simulink model "sampleModel277"  (R2021b)
settings: Solver=VariableStepAuto  StartTime=0.0  StopTime=10.0  RelTol=1e-3
undefined symbols (not defined in the file or in its folder): Newton, Raphson
libraries: simulink x9, slpidlib x1
settings Model: Creator=user  LastModifiedBy=user

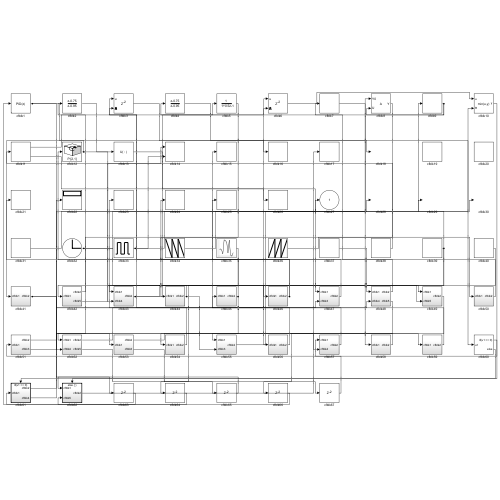
[thumbnail: Simulink's stored preview of the top-level diagram]
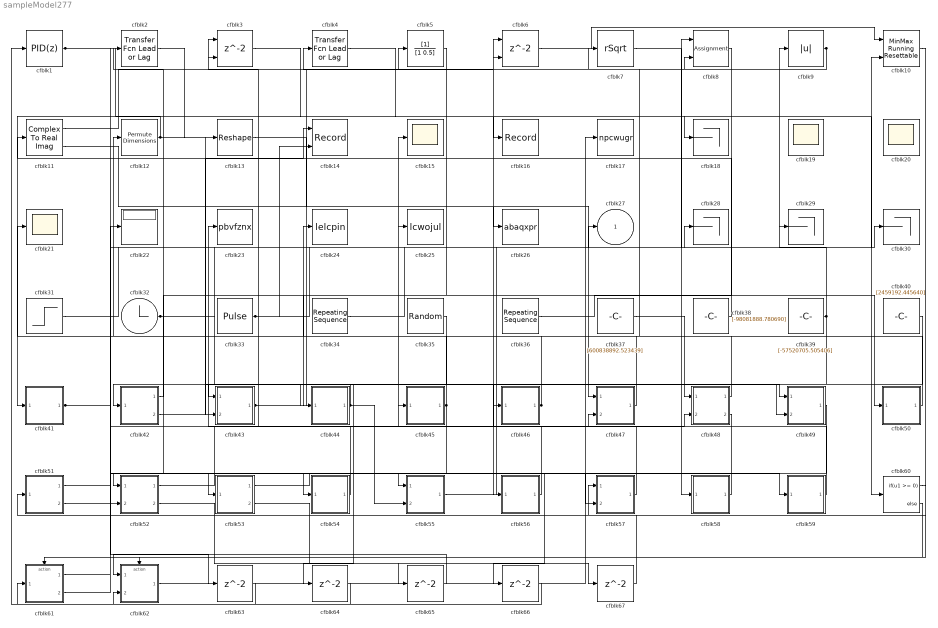
== system sampleModel277 ==
  cfblk1 : slpidlib/PID Controller  Controller=PID  Form=Parallel  TimeDomain=Discrete-time  UseExternalTs=off  SampleTime=1  IntegratorMethod=Forward Euler  FilterMethod=Forward Euler  ControllerParametersSource=internal  P=1  I=1  D=0  UseFilter=on  N=100  TunerSelectOption=Transfer Function Based (PID Tuner App)  InitialConditionSource=internal  InitialConditionForIntegrator=0  InitialConditionForFilter=0  DifferentiatorICPrevScaledInput=0  ExternalReset=none  TrackingMode=off  Kt=1  LimitOutput=off  SatLimitsSource=internal  UpperSaturationLimit=inf  LowerSaturationLimit=-inf  LinearizeAsGain=off  AntiWindupMode=none  Kb=1  POutMin=[]  POutMax=[]  IOutMin=[]  IOutMax=[]  DOutMin=[]  DOutMax=[]  NOutMin=[]  NOutMax=[]  SumOutMin=[]  SumOutMax=[]  SaturationOutMin=[]  SaturationOutMax=[]  PParamMin=[]  PParamMax=[]  IParamMin=[]  IParamMax=[]  DParamMin=[]  DParamMax=[]  NParamMin=[]  NParamMax=[]  KbParamMin=[]  KbParamMax=[]  KtParamMin=[]  KtParamMax=[]  KbOutMin=[]  KbOutMax=[]  KtOutMin=[]  KtOutMax=[]  IntegratorOutMin=[]  IntegratorOutMax=[]  FilterOutMin=[]  FilterOutMax=[]  SumI1OutMin=[]  SumI1OutMax=[]  SumI2OutMin=[]  SumI2OutMax=[]  SumI3OutMin=[]  SumI3OutMax=[]  SumI4OutMin=[]  SumI4OutMax=[]  SumDOutMin=[]  SumDOutMax=[]  DifferentiatorOutMin=[]  DifferentiatorOutMax=[]  FilterDiffOutCoefMin=[]  FilterDiffOutCoefMax=[]  ReciprocalOutMin=[]  ReciprocalOutMax=[]  SumDenOutMin=[]  SumDenOutMax=[]  SumNumOutMin=[]  SumNumOutMax=[]  DivideOutMin=[]  DivideOutMax=[]  UdiffTsProdOutMin=[]  UdiffTsProdOutMax=[]  NTsProdOutMin=[]  NTsProdOutMax=[]  UintegralTsProdOutMin=[]  UintegralTsProdOutMax=[]  UngainTsProdOutMin=[]  UngainTsProdOutMax=[]  IntegratorContinuousStateAttributes=''  IntegratorStateMustResolveToSignalObject=off  IntegratorRTWStateStorageClass=Auto  FilterContinuousStateAttributes=''  FilterStateMustResolveToSignalObject=off  FilterRTWStateStorageClass=Auto  ParallelPVariant=InternalParameters  IdealPVariant=Disabled  IVariant=InternalParameters  DVariant=InternalParameters  IntegratorVariant=Discrete  SatVariant=Disabled  AWVariant=Passthrough  PCopyVariant=Disabled  TRVariant=Disabled  FdbkBlocksVariant=Forward  IdealPFdbkVariant=Disabled  SatFdbkVariant=Disabled  DerivativeFilterVariant=ForwardEulerFilter  NVariant=InternalParameters  NCopyVariant=Disabled  FilterICVariant=InternalICsFilter  IntegratorICVariant=InternalICs  ExternalResetVariant=Disabled  TRSumVariant=Passthrough  SumFdbkVariant=Disabled  SumVariant=Sum_PID  TsampFilterVariant=InternalTs  TsampNgainVariant=Passthrough  TsampIntegralVariant=Passthrough  ExternalSaturationOutDataTypeStr=Inherit: Same as second input
  cfblk10 : simulink/Math Operations/MinMax Running Resettable  Function=min  vinit=0.0
  cfblk11 : ComplexToRealImag
  cfblk12 : PermuteDimensions
  cfblk13 : Reshape
  cfblk14 : Record  FileSettingsInternal="{\"entries\":[{\"content\":{\"excelSettings\":{\"content\":{},\"type\":\"Streamout.ExcelSettings\"}},\"type\":\"Streamout.FileSettingStorage\",\"uuid\":\"d8607e28-881b-4112-add2-e3f322c6c66a\"}],\"packageUris\":[\"http://schema.mathworks.com/mf0/streamout_blocks/R2020a\"],\"version\":\"1.0\"}"  Layout=[1 1]  SignalsInternal="{\"entries\":[{\"content\":{\"signals\":[{\"content\":{\"blockPath\":[\"sampleModel277/cfblk14\"],\"channel\":[],\"dimensions\":[1],\"domain\":\"sampleModel277/cfblk14\",\"lineColor\":\"#a2142f\",\"plots\":[1],\"port\":1,\"sid\":[\"\"],\"signalID\":11589,\"signalName\":\"cfblk42:2\"},\"type\":\"RecordBlkView.Signal\",\"uuid\":\"b47615fb-d819-4e60-bc98-0c25ee9ba6d9\"},{\"content\":{\"blockPath\":[\"sampleModel277/cfblk14\"],\"channel\":[],\"dimensions\":[1],\"domain\":\"sampleModel277/cfblk14\",\"lineColor\":\"#139fff\",\"plots\":[1],\"port\":2,\"sid\":[\"\"],\"signalID\":11593,\"signalName\":\"cfblk33\"},\"type\":\"RecordBlkView.Signal\",\"uuid\":\"1de72bfb-52b8-4dac-a285-8f2b21a8e79d\"}]},\"type\":\"RecordBlkView.InputSignals\",\"uuid\":\"f8287ad3-c409-4800-adb5-27c45d527277\"}],\"packageUris\":[\"http://schema.mathworks.com/mf0/streamout_blocks/R2020a\"],\"version\":\"1.0\"}"  VisualizationBindings="{\"xyplotplugin\":{\"info\":[{\"series\":[{\"bindingParametersList\":[{\"parameter\":\"X-Axis\",\"signalID\":11589,\"signalName\":\"cfblk42:2\"},{\"parameter\":\"Y-Axis\",\"signalID\":11593,\"signalName\":\"cfblk33\"}],\"seriesID\":22106}],\"subplotID\":1}]}}"  CompatibilityTag=XY
  cfblk{15,19..21} (4 alike) : Scope
      cfblk19 settings: Floating=on
      cfblk20 settings: Floating=on
  cfblk16 : Record  FileSettingsInternal="{\"entries\":[{\"content\":{\"excelSettings\":{\"content\":{},\"type\":\"Streamout.ExcelSettings\"}},\"type\":\"Streamout.FileSettingStorage\",\"uuid\":\"0defbab6-1f19-424a-8477-c9e0ae50d269\"}],\"packageUris\":[\"http://schema.mathworks.com/mf0/streamout_blocks/R2020a\"],\"version\":\"1.0\"}"  SignalsInternal="{\"entries\":[{\"content\":{\"signals\":[{\"content\":{\"blockPath\":[\"sampleModel277/cfblk16\"],\"channel\":[],\"dimensions\":[1],\"domain\":\"sampleModel277/cfblk16\",\"lineColor\":\"#ff13a6\",\"plots\":[1],\"port\":1,\"sid\":[\"\"],\"signalID\":11597,\"signalName\":\"cfblk4\"},\"type\":\"RecordBlkView.Signal\",\"uuid\":\"1bcd9140-bb26-4ac9-91fa-95d908c78e84\"}]},\"type\":\"RecordBlkView.InputSignals\",\"uuid\":\"defb70cb-bd16-40b5-b6bd-1390d4c46c9b\"}],\"packageUris\":[\"http://schema.mathworks.com/mf0/streamout_blocks/R2020a\"],\"version\":\"1.0\"}"  VisualizationBindings="{\"sparklinesplugin\":{\"info\":[{\"bindingParametersList\":[],\"subplotID\":1}]}}"
  cfblk17 : ToWorkspace  VariableName=npcwugr  SaveFormat=Timeseries  SampleTime=-1
  cfblk{18,28..30} (4 alike) : Terminator
  cfblk2 : simulink/Discrete/Transfer Fcn Lead or Lag  PoleZ=0.95  ZeroZ=0.75  ICPrevOutput=0.0  ICPrevInput=0.0  DoSatur=off
      settings: SourceProductBaseCode=SL
  cfblk22 : Display
  cfblk23 : ToWorkspace  VariableName=pbvfznx  SaveFormat=Timeseries  SampleTime=-1
  cfblk24 : ToWorkspace  VariableName=lelcpin  SaveFormat=Timeseries  SampleTime=-1
  cfblk25 : ToWorkspace  VariableName=lcwojul  SaveFormat=Timeseries  SampleTime=-1
  cfblk26 : ToWorkspace  VariableName=abaqxpr  SaveFormat=Timeseries  SampleTime=-1
  cfblk3 : Delay  ShowEnablePort=on  SampleTime=1
      settings: InputPortMap=u0,e6
  cfblk31 : Step  Time=[8.000000]  Before=[446463938.940036]  After=[511590212.511346]  SampleTime=0
  cfblk32 : Clock
  cfblk33 : DiscretePulseGenerator  PulseType=Time based  Amplitude=[-336989697.738639]  Period=[82161498.785014]  PulseWidth=5  PhaseDelay=[6.000000]
  cfblk34 : simulink/Sources/Repeating Sequence  rep_seq_t=[0 2]  rep_seq_y=[583198754.923959, 299174869.221675]
  cfblk35 : RandomNumber  Mean=[14216.609925]  Variance=[79975.789287]  Seed=[438589470.000000]  SampleTime=0.1
  cfblk36 : simulink/Sources/Repeating Sequence  rep_seq_t=[0 2]  rep_seq_y=[305355629.704931, 356437179.098536]
  cfblk37 : Constant  Value=[600838892.523439]  SampleTime=1
  cfblk38 : Constant  Value=[-98081888.780690]  SampleTime=1
  cfblk39 : Constant  Value=[-57520705.505406]  SampleTime=1
  cfblk4 : simulink/Discrete/Transfer Fcn Lead or Lag  PoleZ=0.95  ZeroZ=0.75  ICPrevOutput=0.0  ICPrevInput=0.0  DoSatur=off
      settings: SourceProductBaseCode=SL
  cfblk40 : Constant  Value=[2459192.445640]  SampleTime=1
  cfblk41 : Subsystem
  cfblk42 : Subsystem
  cfblk43 : Subsystem
  cfblk44 : Subsystem
  cfblk45 : Subsystem
  cfblk46 : Subsystem
  cfblk47 : Subsystem
  cfblk48 : Subsystem
  cfblk49 : Subsystem
  cfblk5 : DiscreteFilter  SampleTime=1
  cfblk50 : Subsystem
  cfblk51 : Subsystem
  cfblk52 : Subsystem
  cfblk53 : Subsystem
  cfblk54 : Subsystem
  cfblk55 : Subsystem
  cfblk56 : Subsystem
  cfblk57 : Subsystem
  cfblk58 : Subsystem
  cfblk59 : Subsystem
  cfblk6 : Delay  ShowEnablePort=on  SampleTime=1
      settings: InputPortMap=u0,e6
  cfblk60 : If  IfExpression=u1 >= 0  SampleTime=1
  cfblk61 : Subsystem  TreatAsAtomicUnit=on
  cfblk62 : Subsystem  TreatAsAtomicUnit=on
  cfblk{63..67} (5 alike) : Delay  SampleTime=1
  cfblk7 : Sqrt  Operator=rSqrt  AlgorithmType=Newton-Raphson  SaturateOnIntegerOverflow=on
  cfblk8 : Assignment  DiagnosticForDimensions=Warning  IndexOptions=Index vector (dialog)  Indices=1  OutputSizes=1
  cfblk9 : Abs
  cfblk27 : Outport
  wires:
  cfblk53/1(cfblk2) -> cfblk59/1(cfblk1)
  cfblk48/1(cfblk2) -> cfblk12/1
  cfblk44/1(cfblk2) -> cfblk42/1(cfblk1), cfblk55/2(cfblk3)
  cfblk2/1 -> cfblk13/1
  cfblk54/1(cfblk2) -> cfblk23/1
  cfblk36/1 -> cfblk50/1(cfblk1)
  cfblk6/1 -> cfblk10/1
  cfblk9/1 -> cfblk4/1, cfblk8/2
  cfblk10/1 -> cfblk57/1(cfblk1)
  cfblk12/1 -> cfblk41/1(cfblk1), cfblk49/2(cfblk5)
  cfblk11/1 -> cfblk6/1
  cfblk43/1(cfblk2) -> cfblk5/1, cfblk49/1(cfblk1)
  cfblk31/1 -> cfblk9/1
  cfblk58/1(cfblk2) -> cfblk55/1(cfblk1)
  cfblk40/1 -> cfblk43/1(cfblk1)
  cfblk11/2 -> cfblk47/1(cfblk1)
  cfblk52/1(cfblk2) -> cfblk6/2
  cfblk38/1 -> cfblk11/1
  cfblk35/1 -> cfblk43/2(cfblk4)
  cfblk1/1 -> cfblk60/1, cfblk57/2(cfblk4)
  cfblk13/1 -> cfblk26/1
  cfblk39/1 -> cfblk29/1, cfblk54/1(cfblk1), cfblk46/1(cfblk1)
  cfblk55/1(cfblk2) -> cfblk28/1
  cfblk62/1(cfblk2) -> cfblk17/1
  cfblk3/1 -> cfblk18/1
  cfblk59/1(cfblk2) -> cfblk15/1
  cfblk34/1 -> cfblk30/1
  cfblk33/1 -> cfblk10/2, cfblk14/2
  cfblk50/1(cfblk2) -> cfblk7/1
  cfblk41/1(cfblk2) -> cfblk47/2(cfblk3), cfblk63/1
  cfblk42/1(cfblk2) -> cfblk2/1
  cfblk45/1(cfblk2) -> cfblk25/1, cfblk64/1
  cfblk57/1(cfblk2) -> cfblk45/1(cfblk1)
  cfblk37/1 -> cfblk48/1(cfblk1)
  cfblk32/1 -> cfblk56/1(cfblk1), cfblk8/1
  cfblk8/1 -> cfblk44/1(cfblk1)
  cfblk5/1 -> cfblk52/1(cfblk1)
  cfblk49/1(cfblk2) -> cfblk52/2(cfblk4)
  cfblk7/1 -> cfblk58/1(cfblk1)
  cfblk47/1(cfblk2) -> cfblk24/1
  cfblk46/1(cfblk2) -> cfblk21/1, cfblk3/2
  cfblk56/1(cfblk2) -> cfblk3/1
  cfblk4/1 -> cfblk16/1
  cfblk51/1(cfblk2) -> cfblk53/1(cfblk1)
  cfblk42/2(cfblk5) -> cfblk14/1
  cfblk51/2(cfblk3) -> cfblk22/1
  cfblk61/1(cfblk2) -> cfblk27/1
  cfblk61/2(cfblk4) -> cfblk48/2(cfblk4)
  cfblk60/1 -> cfblk61/Action
  cfblk60/2 -> cfblk62/Action
  cfblk63/1 -> cfblk1/1
  cfblk64/1 -> cfblk61/1(cfblk1)
  cfblk52/2(cfblk5) -> cfblk65/1
  cfblk65/1 -> cfblk62/1(cfblk1)
  cfblk48/2(cfblk5) -> cfblk66/1
  cfblk66/1 -> cfblk62/2(cfblk5)
  cfblk53/2(cfblk3) -> cfblk67/1
  cfblk67/1 -> cfblk51/1(cfblk1)

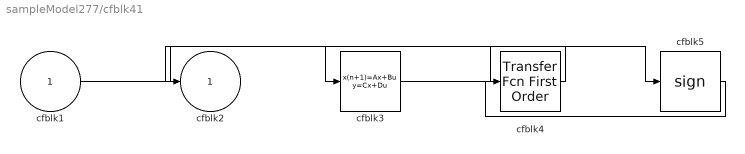
== system sampleModel277/cfblk41 ==
  cfblk1 : Inport
  cfblk3 : DiscreteStateSpace
  cfblk4 : simulink/Discrete/Transfer Fcn First Order  PoleZ=0.95  ICPrevOutput=0.0  DoSatur=off
  cfblk5 : Signum
  cfblk2 : Outport
  wires:
  cfblk3/1 -> cfblk5/1
  cfblk5/1 -> cfblk4/1
  cfblk1/1 -> cfblk3/1
  cfblk4/1 -> cfblk2/1

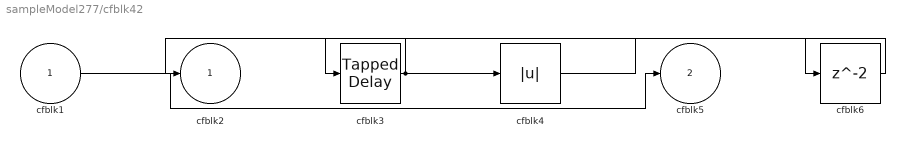
== system sampleModel277/cfblk42 ==
  cfblk1 : Inport
  cfblk3 : simulink/Discrete/Tapped Delay  vinit=0.0  samptime=-1  NumDelays=1  DelayOrder=Oldest  includeCurrent=off
  cfblk4 : Abs
  cfblk6 : Delay  SampleTime=1
  cfblk2 : Outport
  cfblk5 : Outport  Port=2
  wires:
  cfblk3/1 -> cfblk4/1, cfblk2/1
  cfblk1/1 -> cfblk5/1
  cfblk4/1 -> cfblk6/1
  cfblk6/1 -> cfblk3/1

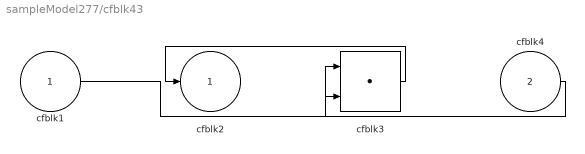
== system sampleModel277/cfblk43 ==
  cfblk1 : Inport
  cfblk4 : Inport  Port=2
  cfblk3 : DotProduct  InputSameDT=on  OutDataTypeStr=Inherit: Inherit via internal rule
  cfblk2 : Outport
  wires:
  cfblk3/1 -> cfblk2/1
  cfblk4/1 -> cfblk3/1
  cfblk1/1 -> cfblk3/2

== system sampleModel277/cfblk44 ==
  cfblk1 : Inport
  cfblk3 : DiscreteZeroPole  Poles=[0 0.5]  Gain=1
  cfblk2 : Outport
  wires:
  cfblk1/1 -> cfblk3/1
  cfblk3/1 -> cfblk2/1

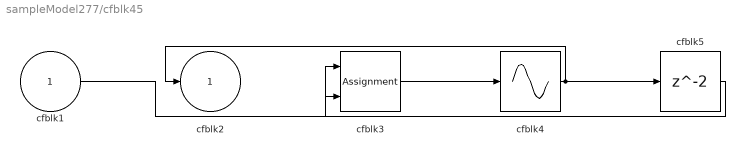
== system sampleModel277/cfblk45 ==
  cfblk1 : Inport
  cfblk3 : Assignment  DiagnosticForDimensions=Warning  IndexOptions=Index vector (dialog)  Indices=1  OutputSizes=1
  cfblk4 : Sin  TimeSource=Use external signal  SampleTime=0
  cfblk5 : Delay  SampleTime=1
  cfblk2 : Outport
  wires:
  cfblk4/1 -> cfblk2/1, cfblk5/1
  cfblk3/1 -> cfblk4/1
  cfblk1/1 -> cfblk3/1
  cfblk5/1 -> cfblk3/2

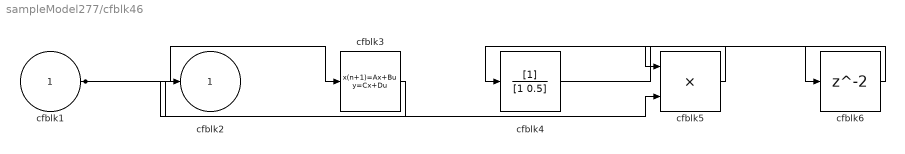
== system sampleModel277/cfblk46 ==
  cfblk1 : Inport
  cfblk3 : DiscreteStateSpace
  cfblk4 : DiscreteFilter  SampleTime=1
  cfblk5 : Product
  cfblk6 : Delay  SampleTime=1
  cfblk2 : Outport
  wires:
  cfblk5/1 -> cfblk4/1
  cfblk1/1 -> cfblk3/1, cfblk5/2
  cfblk3/1 -> cfblk2/1
  cfblk4/1 -> cfblk6/1
  cfblk6/1 -> cfblk5/1

== system sampleModel277/cfblk47 ==
  cfblk1 : Inport
  cfblk3 : Inport  Port=2
  cfblk2 : Outport
  wires:
  cfblk1/1 -> cfblk2/1

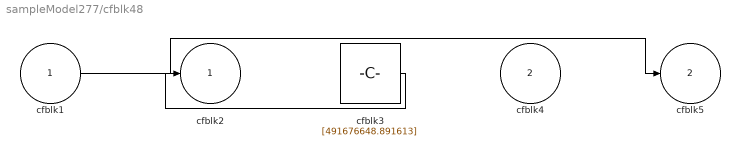
== system sampleModel277/cfblk48 ==
  cfblk1 : Inport
  cfblk4 : Inport  Port=2
  cfblk3 : Constant  Value=[491676648.891613]  SampleTime=1
  cfblk2 : Outport
  cfblk5 : Outport  Port=2
  wires:
  cfblk1/1 -> cfblk5/1
  cfblk3/1 -> cfblk2/1

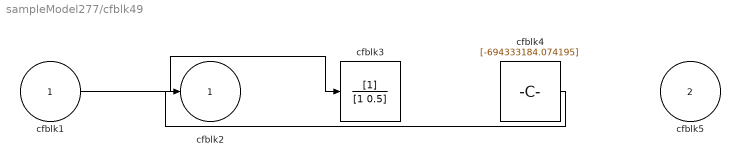
== system sampleModel277/cfblk49 ==
  cfblk1 : Inport
  cfblk5 : Inport  Port=2
  cfblk3 : DiscreteFilter  SampleTime=1
  cfblk4 : Constant  Value=[-694333184.074195]  SampleTime=1
  cfblk2 : Outport
  wires:
  cfblk1/1 -> cfblk3/1
  cfblk4/1 -> cfblk2/1

== system sampleModel277/cfblk50 ==
  cfblk1 : Inport
  cfblk3 : Sin  TimeSource=Use external signal  SampleTime=0
  cfblk2 : Outport
  wires:
  cfblk1/1 -> cfblk2/1, cfblk3/1

== system sampleModel277/cfblk51 ==
  cfblk1 : Inport
  cfblk2 : Outport
  cfblk3 : Outport  Port=2
  wires:
  cfblk1/1 -> cfblk2/1, cfblk3/1

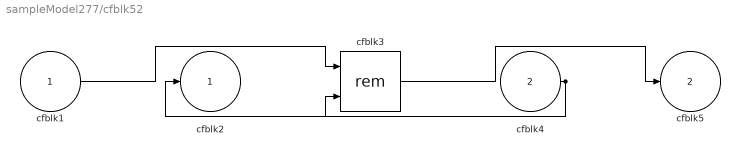
== system sampleModel277/cfblk52 ==
  cfblk1 : Inport
  cfblk4 : Inport  Port=2
  cfblk3 : Math  Operator=rem  SaturateOnIntegerOverflow=on
  cfblk2 : Outport
  cfblk5 : Outport  Port=2
  wires:
  cfblk3/1 -> cfblk5/1
  cfblk4/1 -> cfblk2/1, cfblk3/2
  cfblk1/1 -> cfblk3/1

== system sampleModel277/cfblk53 ==
  cfblk1 : Inport
  cfblk2 : Outport
  cfblk3 : Outport  Port=2
  wires:
  cfblk1/1 -> cfblk2/1, cfblk3/1

== system sampleModel277/cfblk54 ==
  cfblk1 : Inport
  cfblk3 : DiscreteTransferFcn  SampleTime=1
  cfblk2 : Outport
  wires:
  cfblk1/1 -> cfblk3/1
  cfblk3/1 -> cfblk2/1

== system sampleModel277/cfblk55 ==
  cfblk1 : Inport
  cfblk3 : Inport  Port=2
  cfblk2 : Outport
  wires:
  cfblk3/1 -> cfblk2/1

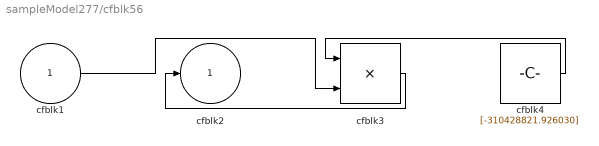
== system sampleModel277/cfblk56 ==
  cfblk1 : Inport
  cfblk3 : Product  Inputs=**
  cfblk4 : Constant  Value=[-310428821.926030]  SampleTime=1
  cfblk2 : Outport
  wires:
  cfblk4/1 -> cfblk3/1
  cfblk3/1 -> cfblk2/1
  cfblk1/1 -> cfblk3/2

== system sampleModel277/cfblk57 ==
  cfblk1 : Inport
  cfblk4 : Inport  Port=2
  cfblk3 : MinMax  Function=max  Inputs=3
  cfblk2 : Outport
  wires:
  cfblk1/1 -> cfblk2/1
  cfblk4/1 -> cfblk3/1, cfblk3/2, cfblk3/3

== system sampleModel277/cfblk58 ==
  cfblk1 : Inport
  cfblk3 : Signum
  cfblk2 : Outport
  wires:
  cfblk1/1 -> cfblk2/1, cfblk3/1

== system sampleModel277/cfblk59 ==
  cfblk1 : Inport
  cfblk3 : simulink/Discrete/Tapped Delay  vinit=0.0  samptime=-1  NumDelays=1  DelayOrder=Oldest  includeCurrent=off
  cfblk4 : Constant  Value=[966953148.697981]  SampleTime=1
  cfblk2 : Outport
  wires:
  cfblk3/1 -> cfblk2/1
  cfblk4/1 -> cfblk3/1

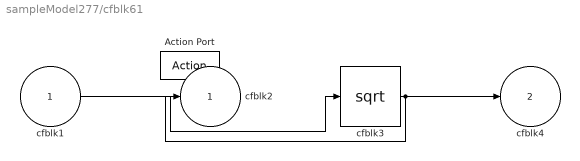
== system sampleModel277/cfblk61 ==
  cfblk1 : Inport
  Action Port : ActionPort  ActionPortLabel=if(u1 >= 0)
  cfblk3 : Sqrt  SaturateOnIntegerOverflow=on
  cfblk2 : Outport
  cfblk4 : Outport  Port=2
  wires:
  cfblk1/1 -> cfblk3/1
  cfblk3/1 -> cfblk2/1, cfblk4/1

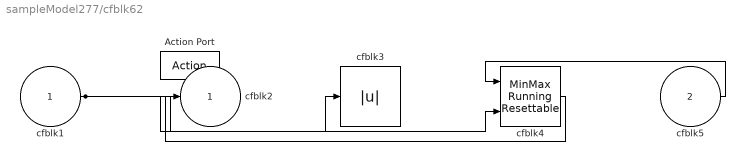
== system sampleModel277/cfblk62 ==
  cfblk1 : Inport
  cfblk5 : Inport  Port=2
  Action Port : ActionPort  ActionPortLabel=else
  cfblk3 : Abs
  cfblk4 : simulink/Math Operations/MinMax Running Resettable  Function=min  vinit=0.0
  cfblk2 : Outport
  wires:
  cfblk5/1 -> cfblk4/1
  cfblk1/1 -> cfblk4/2, cfblk3/1
  cfblk4/1 -> cfblk2/1
